simulink model "regulator_LQG"  (Simulink 10.0)
settings: Solver=ode45  StartTime=0.0  StopTime=tsim  RelTol=1e-3  EnableMultiTasking=on
values from neighbouring files (symbols this model uses):
  B_noise = [B ones(size(B,1),1)]    [es2.m]
  C_states = eye(2)    [es2.m]
  D_noise = [D_states zeros(size(D_states,1),1)]    [es2.m]
  Klqr1 = lqr(A,B,Q,R)    [es2.m]
  NK = 0    [es2.m]
  RK = QK(1)*100    [es2.m]
  sat_max = inf    [es2.m]
  sat_min = -inf    [es2.m]
  x0 = [0 10]    [es2.m]
  x0K = 1.5*x0    [es2.m]
undefined symbols (not defined in the file or in its folder): A, B, C, Continuous, D, Time
libraries: simulink x2, ctrlSharedLib x1
settings Model: Creator=Administrator  LastModifiedBy=Chiara
settings DataIOCC: LimitDataPoints=on  SignalLoggingSaveFormat=ModelDataLogs
settings OptimizationCC: ExpressionDepthLimit=2147483647  InitFltsAndDblsToZero=on
settings DebuggingCC: SolverPrmCheckMsg=warning  FcnCallInpInsideContextMsg=warning  StateNameClashWarn=warning
settings GRTTargetCC: GeneratePreprocessorConditionals=Disable all
settings ConfigComp: CovExternalEMLEnable=off  CovSFcnEnable=off

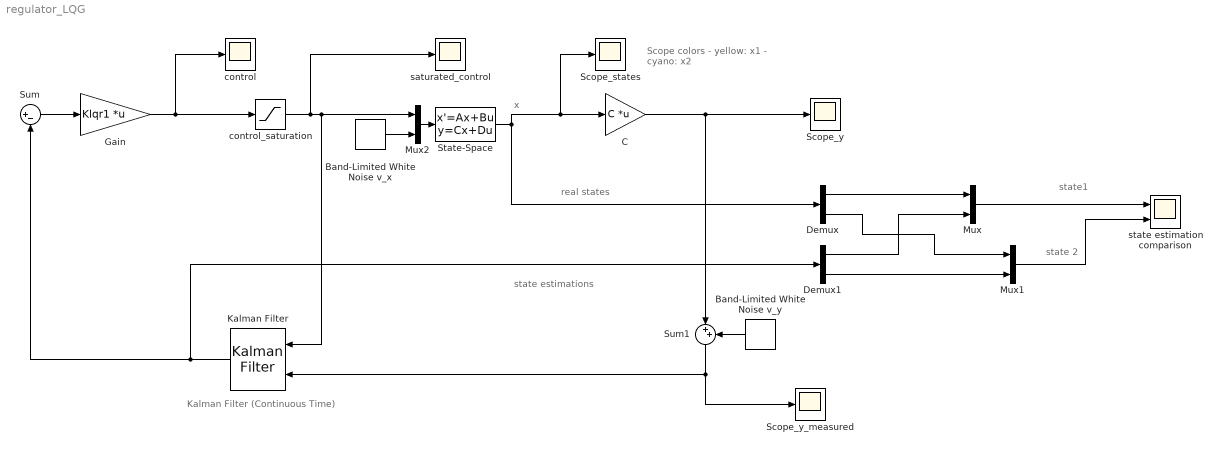
== system regulator_LQG ==
  note: Kalman Filter (Continuous Time)
  note: state 2
  note: state1
  note: real states
  note: state estimations
  note: x
  note: Scope colors
      | - yellow: x1
      | - cyano: x2
  "Band-Limited White Noise v_x   " : simulink/Sources/Band-Limited White Noise  Cov=power_vx  Ts=0.1  seed=[23341]
  Band-Limited White Noise v_y : simulink/Sources/Band-Limited White Noise  Cov=power_vy  Ts=0.1  seed=[1258]
  C : Gain  Gain=C  Multiplication=Matrix(K*u)
  Demux : Demux  Outputs=2
  Demux1 : Demux  Outputs=2
  Gain : Gain  Gain=Klqr1  Multiplication=Matrix(K*u)
  Kalman Filter : ctrlSharedLib/Kalman Filter  TimeDomain=Continuous-Time  UseCurrentEstimator=on  ModelSource=Individual A, B, C, D matrices  ModelSourceVariable=ss(0.95,1,1,0,1)  A=A  B=B  C=C  D=D  NumberOfStates=1  NumberOfInputs=1  NumberOfOutputs=1  InitialEstimateSource=Dialog  X0=x0K  P0=10  UseK=off  UseGH=off  NumberOfProcessNoiseInputs=1  G=1  TimeInvariantG=on  H=0  TimeInvariantH=on  Q=QK  TimeInvariantQ=on  R=RK  TimeInvariantR=on  N=NK  TimeInvariantN=on  AddInputPort=on  AddEnablePort=off  OutputEstimatedY=off  OutputP=off  Ts=-1
      settings: SourceProductBaseCode=CT
  Mux : Mux  Inputs=2
  Mux1 : Mux  Inputs=2
  Mux2 : Mux  Inputs=2
  Scope_states : Scope
  Scope_y : Scope
  Scope_y_measured : Scope
  "State-Space " : StateSpace  A=A  B=B_noise  C=C_states  D=D_noise  InitialCondition=x0
  Sum : Sum  Inputs=|+-
  Sum1 : Sum  Inputs=|++
  control : Scope
  control_saturation : Saturate  UpperLimit=sat_max  LowerLimit=sat_min
  saturated_control : Scope
  "state estimation comparison  " : Scope  NumInputPorts=2
  wires:
  Gain/1 -> control_saturation/1, control/1
  Sum/1 -> Gain/1
  "State-Space "/1 -> Scope_states/1, C/1, Demux/1
  C/1 -> Sum1/1, Scope_y/1
  control_saturation/1 -> Mux2/1, Kalman Filter/1, saturated_control/1
  Kalman Filter/1 -> Demux1/1, Sum/2
  Demux/1 -> Mux/1
  Demux1/1 -> Mux/2
  Demux1/2 -> Mux1/2
  Demux/2 -> Mux1/1
  Mux1/1 -> "state estimation comparison  "/2
  Mux/1 -> "state estimation comparison  "/1
  Mux2/1 -> "State-Space "/1
  Sum1/1 -> Scope_y_measured/1, Kalman Filter/2
  Band-Limited White Noise v_y/1 -> Sum1/2
  "Band-Limited White Noise v_x   "/1 -> Mux2/2
